simulink model "CCCV_v3"  (R2019a)
settings: Solver=FixedStepAuto  StartTime=0.0  StopTime=10000  FixedStep=1  RelTol=1e-3
values from neighbouring files (symbols this model uses):
  x0_nom = [97.2776595046 97.2776595046 97.2776595046 97.2776595046 97.2776595046 97.2776595046 97.2776595046 97.2776595046 97.2776595046 97.2776595046 97.2776595046 97.2776595046 ... (83 elements, 83x1)]    [x0_nom.mat]
settings Model: Creator=ztakeo  LastModifiedBy=ztakeo

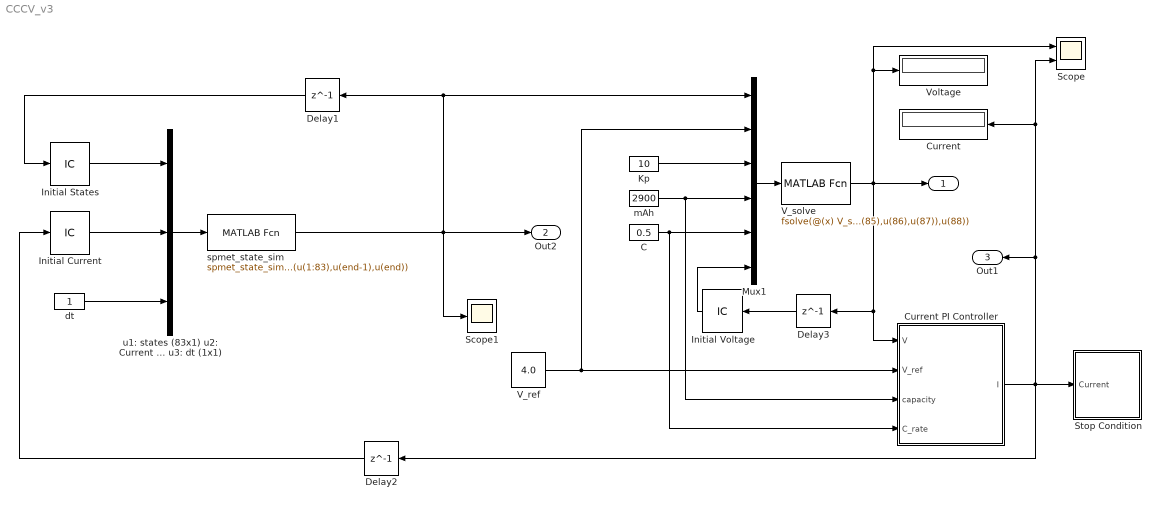
== system CCCV_v3 ==
  C : Constant  Value=0.5
  Current : Display
  Current PI Controller : MATLAB Function  TreatAsAtomicUnit=on
  Delay1 : Delay  DelayLength=1  InitialCondition=0
  Delay2 : Delay  DelayLength=1  InitialCondition=0
  Delay3 : Delay  DelayLength=1  InitialCondition=0
  Initial Current : InitialCondition  Value=0
  "Initial States " : InitialCondition  Value=x0_nom
  "Initial Voltage " : InitialCondition  Value=2.8
  Kp : Constant  Value=10
  Mux1 : Mux  Inputs=6
  Scope : Scope  NumInputPorts=2
  Scope1 : Scope
  Stop Condition : Subsystem
  "V_ref " : Constant  Value=4.0
  V_solve : MATLABFcn  MATLABFcn=fsolve(@(x) V_solve(x, u(1:83), u(84),u(85),u(86),u(87)),u(88))  OutputDimensions=1
  "Voltage " : Display
  dt : Constant
  mAh : Constant  Value=2900
  spmet_state_sim : MATLABFcn  MATLABFcn=spmet_state_sim(u(1:83),u(end-1),u(end))  OutputDimensions=83  OutputSignalType=real
  "u1: states (83x1) u2: Current (1x1) u3: dt (1x1) " : Mux  Inputs=3
  " " : Outport  SignalName=V
  Out2 : Outport  Port=2  SignalName=x
  Out1 : Outport  Port=3  SignalName=Current
  wires:
  spmet_state_sim/1 -> Mux1/1, Delay1/1, Out2/1, Scope1/1
  Delay3/1 -> "Initial Voltage "/1
  Delay1/1 -> "Initial States "/1
  Current PI Controller/1(I) -> Scope/2, Current/1, Out1/1, Stop Condition/1(Current), Delay2/1
  Mux1/1 -> V_solve/1
  Initial Current/1 -> "u1: states (83x1) u2: Current (1x1) u3: dt (1x1) "/2
  "V_ref "/1 -> Current PI Controller/2(V_ref), Mux1/2
  mAh/1 -> Mux1/4, Current PI Controller/3(capacity)
  Delay2/1 -> Initial Current/1
  "u1: states (83x1) u2: Current (1x1) u3: dt (1x1) "/1 -> spmet_state_sim/1
  V_solve/1 -> Delay3/1, Current PI Controller/1(V), " "/1, Scope/1, "Voltage "/1
  C/1 -> Mux1/5, Current PI Controller/4(C_rate)
  "Initial States "/1 -> "u1: states (83x1) u2: Current (1x1) u3: dt (1x1) "/1
  "Initial Voltage "/1 -> Mux1/6
  Kp/1 -> Mux1/3
  dt/1 -> "u1: states (83x1) u2: Current (1x1) u3: dt (1x1) "/3

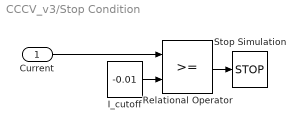
== system CCCV_v3/Stop Condition ==
  Current : Inport
  I_cutoff : Constant  Value=-0.01
  Relational Operator : RelationalOperator  OutDataTypeStr=boolean  RndMeth=Simplest
  Stop Simulation : Stop
  wires:
  Current/1 -> Relational Operator/1
  Relational Operator/1 -> Stop Simulation/1
  I_cutoff/1 -> Relational Operator/2

== matlab function CCCV_v3/Current PI Controller ==
  data: V input; V_ref input; I output; capacity input; C_rate input
%% PI Controller function
function I = fcn(V,V_ref,capacity,C_rate)
    I_chrgmax = -capacity*C_rate/1000; %A

    Kp = 10;
    
    % Compute control law current, but regulate if above max charge rate
    I_ctrl = Kp*(V-V_ref);
    
    if I_ctrl < I_chrgmax % charging current is negative, so higher charging rate is a more negative value
        scale_Kp = I_chrgmax/I_ctrl; % bound the max current; here use max instead of min because charge current is (-)
        % recompute Kp if         
        I = scale_Kp*Kp*(V-V_ref);
    else % case where charging current from controller doesn't exceed max rate
        I = I_ctrl;
    end

end
